simulink model "sm_car_testrig_bus_VehBusBody"  (R2020b)
settings: Solver=VariableStepAuto  StartTime=0.0  StopTime=10.0  RelTol=1e-3
libraries: sm_car_lib x2, sm_lib x2, nesl_utility x1
Description:
  | Copyright 2020 The MathWorks, Inc.
settings Model: Creator=smiller  LastModifiedBy=smiller
settings DataIOCC: ReturnWorkspaceOutputs=off
settings DebuggingCC: ArithmeticOperatorsInVariantConditions=warning
settings SFSimCC: CustomCodeUndefinedFunction=UseInterfaceOnly
settings DiagnosticsConfigSet: SimMechanicsConflictingReferenceFrames=none
settings ExplorerConfigSet: SimMechanicsOpenEditorOnUpdate=off

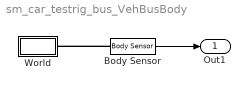
== system sm_car_testrig_bus_VehBusBody ==
  Body Sensor : sm_car_lib/Sensors/Body Sensor  offset_body_sensor=Vehicle.Chassis.Body.sCG.Value
  World : Subsystem
      mask Display: disp('Wld')
  Out1 : Outport  OutDataTypeStr=Bus: VehicleBodyBusDef  VectorParamsAs1DForOutWhenUnconnected=off
      settings: AttributesFormatString=%<OutDataTypeStr>
  wires:
  Body Sensor/1 -> Out1/1
  connections:
  Body Sensor/LConn1 -- World/RConn1

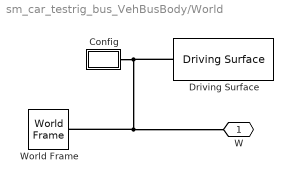
== system sm_car_testrig_bus_VehBusBody/World ==
  Config : Subsystem
  Driving Surface : sm_car_lib/Environment/Driving Surface  LabelModeActiveChoice=Floor_Grid
  World Frame : sm_lib/Frames and Transforms/World Frame
  W : PMIOPort  Side=Right
  connections:
  Config/RConn1 -- Driving Surface/RConn1 -- World Frame/RConn1 -- W/RConn1

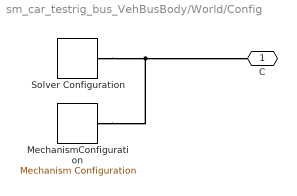
== system sm_car_testrig_bus_VehBusBody/World/Config ==
  MechanismConfiguration : sm_lib/Utilities/Mechanism Configuration  UniformGravity=Constant  GravityVector=[0 0 -9.80665]  GravityVectorUnits=m/s^2  GravityUnits=m/s^2  LinearizationDelta=0.001  JointModeTransitionNonlinearIterations=2
  Solver Configuration : nesl_utility/Solver Configuration  PhysicalDomain=network_engine_domain  SubClassName=solver  LeftPortType=input  RightPortType=generic  Tones=[]  Harmonics=[]  SimulateNoise=off  Profile=off  UseLocalSampling=off  EnableSwitchedLinearOptims=on  FrequencyDomain=off  UseCCode=off  RelTol=0.001  AbsTol=1e-06  MinStep=1e-09  ToWorkspace=off  RevertToSquareIcSolve=off  NumHomotopyIterations=100  PhasorMode=off  PhasorModeNumHarmonics=1  DoDC=off  ResidualTolerance=1e-9  UseLocalSolver=off  LocalSolverChoice=NE_BACKWARD_EULER_ADVANCER  LocalSolverSampleTime=0.00025*4  DoFixedCost=off  MaxNonlinIter=3  MaxModeIter=2  ComputeImpulses=off  ImpulseIterations=2  LinearAlgebra=Sparse  EquationFormulation=NE_TIME_EF  DelaysMemoryBudget=1024  AutomaticFiltering=on  FilteringTimeConstant=0.001  PartitionStorageMethod=AS_NEEDED  PartitionMemoryBudget=1024  PartitionMethod=FAST
  C : PMIOPort  Side=Right
  connections:
  Solver Configuration/RConn1 -- C/RConn1 -- MechanismConfiguration/RConn1
